simulink model "transversal_model"  (R2023b)
settings: Solver=FixedStepDiscrete  StartTime=0.0  StopTime=0.01  RelTol=1e-3
undefined symbols (not defined in the file): mf1, mf2, mf3, mfIdeal, pw
libraries: phaseddetectlib x9, phasedenvlib x4, phasedtxrxlib x2, dspfdesign x1, phasedwavlib x1
settings Model: Creator=krsh  LastModifiedBy=krsh
settings SolverCC: AlgebraicLoopSolver=TrustRegion  AutoInsertRateTranBlk=on
settings DataIOCC: LimitDataPoints=on  SaveOutput=off  SignalLogging=off  SaveTime=off
settings OptimizationCC: ReuseModelBlockBuffer=off  LifeSpan=inf  SimCompilerOptimization=on
settings DebuggingCC: AlgebraicLoopMsg=error  SingleTaskRateTransMsg=error  UnconnectedInputMsg=warning  UnconnectedOutputMsg=warning  UnconnectedLineMsg=warning  AllowSymbolicDim=off  SubsystemReferenceDiagnosticForUnitTest=warning  SFUnexpectedBacktrackingDiag=warning  SFNoUnconditionalDefaultTransitionDiag=warning  SFExecutionAtInitializationDiag=none  ArithmeticOperatorsInVariantConditions=warning
settings ModelReferenceCC: EnableRefExpFcnMdlSchedulingChecks=on
settings SFSimCC: SimUseLocalCustomCode=off  CustomCodeUndefinedFunction=UseInterfaceOnly
settings RTWCC: RTWUseLocalCustomCode=off
settings CodeAppCC: StateflowObjectComments=on
settings GRTTargetCC: TargetLangStandard=C89/C90 (ANSI)
settings ConfigComp: CovMetricSettings=dw  CovSaveCumulativeToWorkspaceVar=on  CovSaveSingleToWorkspaceVar=on  CovExternalEMLEnable=off  CovSFcnEnable=off

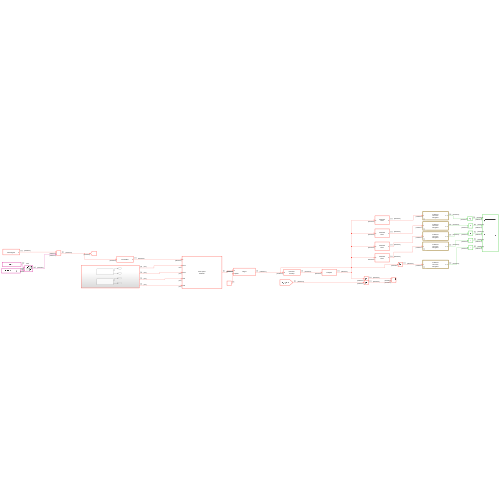
[thumbnail: Simulink's stored preview of the top-level diagram]
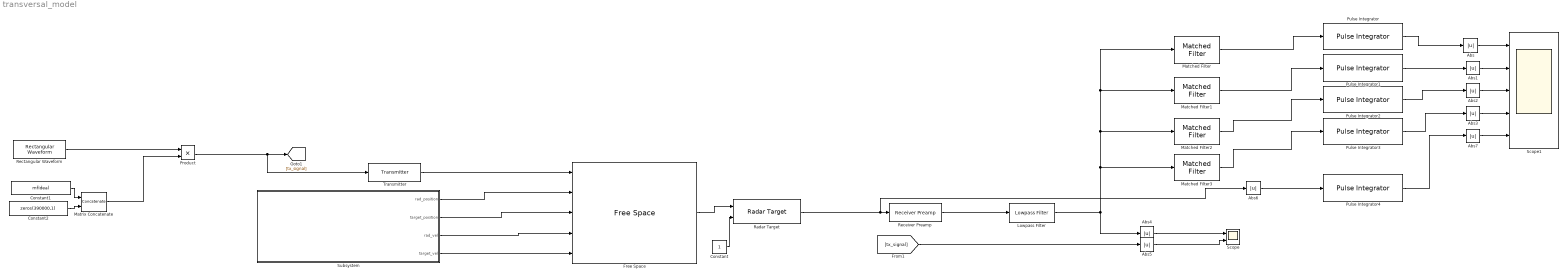
== system transversal_model ==
  Abs{,1..7} (8 alike) : Abs  SaturateOnIntegerOverflow=off
  Constant : Constant  SampleTime=-1
  Constant1 : Constant  Value=mfIdeal
  Constant2 : Constant  Value=zeros(390000,1)
  Free Space : phasedenvlib/Free Space  PropagationSpeed=c  OperatingFrequency=3e8  TwoWayPropagation=off  SampleRateFromInputCheckbox=on  SampleRate=1e6  MaximumDistanceSource=Property  MaximumDistance=2e3  MaximumNumInputSamplesSource=Auto  MaximumNumInputSamples=1000  SimulateUsing=Interpreted execution
  Lowpass Filter : dspfdesign/Lowpass Filter  FilterType=IIR  DesignForMinimumOrder=off  FilterOrder=3  PassbandFrequency=pulse_bw  StopbandFrequency=12e3  PassbandRipple=0.1  StopbandAttenuation=80  SampleRateMode=Specify on dialog  SampleRate=fs  SimulateUsing=Interpreted execution  roundingMode=Floor  coeffsDataTypeStr=fixdt(1,16)
  Matched Filter : phaseddetectlib/Matched Filter  CoefficientsSource=Property  Coefficients=mfIdeal'  SpectrumWindow=None  CustomSpectrumWindow=@hamming  SpectrumRange=[ 0, 1e5 ]  SampleRateFromInputCheckbox=on  SampleRate=1e6  SidelobeAttenuation=30  Beta=0.5  Nbar=4  GainOutputPort=off  MaximumNumInputSamplesSource=Auto  MaximumNumInputSamples=100  SimulateUsing=Interpreted execution
  Matched Filter1 : phaseddetectlib/Matched Filter  CoefficientsSource=Property  Coefficients=mf1.coeffs.Numerator'  SpectrumWindow=None  CustomSpectrumWindow=@hamming  SpectrumRange=[ 0, 1e5 ]  SampleRateFromInputCheckbox=on  SampleRate=1e6  SidelobeAttenuation=30  Beta=0.5  Nbar=4  GainOutputPort=off  MaximumNumInputSamplesSource=Auto  MaximumNumInputSamples=100  SimulateUsing=Interpreted execution
  Matched Filter2 : phaseddetectlib/Matched Filter  CoefficientsSource=Property  Coefficients=mf2.coeffs.Numerator'  SpectrumWindow=None  CustomSpectrumWindow=@hamming  SpectrumRange=[ 0, 1e5 ]  SampleRateFromInputCheckbox=on  SampleRate=1e6  SidelobeAttenuation=30  Beta=0.5  Nbar=4  GainOutputPort=off  MaximumNumInputSamplesSource=Auto  MaximumNumInputSamples=100  SimulateUsing=Interpreted execution
  Matched Filter3 : phaseddetectlib/Matched Filter  CoefficientsSource=Property  Coefficients=mf3.coeffs.Numerator'  SpectrumWindow=None  CustomSpectrumWindow=@hamming  SpectrumRange=[ 0, 1e5 ]  SampleRateFromInputCheckbox=on  SampleRate=1e6  SidelobeAttenuation=30  Beta=0.5  Nbar=4  GainOutputPort=off  MaximumNumInputSamplesSource=Auto  MaximumNumInputSamples=100  SimulateUsing=Interpreted execution
  Matrix Concatenate : Concatenate  Mode=Multidimensional array
  Product : Product
  Pulse Integrator{,1..4} (5 alike) : phaseddetectlib/Pulse Integrator  CoherentFlag=Coherent  N=10  V=0
  Radar Target : phasedenvlib/Radar Target  EnablePolarization=off  Mode=Monostatic  MeanRCSSource=Property  ScatteringMatrixSource=Property  MeanRCS=1  ScatteringMatrix=eye( 2 )  Model=Swerling1  PropagationSpeed=c  OperatingFrequency=3e8  SeedSource=Auto  Seed=0  SimulateUsing=Interpreted execution
  Receiver Preamp : phasedtxrxlib/Receiver Preamp  Gain=3  LossFactor=0  NoiseMethod=Noise power  NoiseFigure=1.2  ReferenceTemperature=290  SampleRateFromInputCheckbox=on  SampleRate=1e6  NoisePower=0.002  EnableInputPort=off  PhaseNoiseInputPort=off  SeedSource=Auto  Seed=0  SimulateUsing=Interpreted execution
  Rectangular Waveform : phasedwavlib/Rectangular Waveform  SampleRate=fs  DurationSpecification=Pulse width  PulseWidth=pw  DutyCycle=0.5  PRF=prf  PRFSelectionInputPort=off  SimulationTimeSource=Derive from waveform parameters  FrequencyOffsetSource=Property  FrequencyOffset=0  OutputFormat=Pulses  NumSamples=100  NumPulses=1  PRFOutputPort=off  CoefficientsOutputPort=off  SimulateUsing=Interpreted execution
  Scope : Scope  NumInputPorts=2
  Scope1 : Scope  NumInputPorts=5
  Subsystem : Subsystem
  Transmitter : phasedtxrxlib/Transmitter  PeakPower=tx_peak_power  Gain=13  LossFactor=0  InUseOutputPort=off  CoherentOnTransmit=on  PhaseNoiseOutputPort=off  SeedSource=Auto  Seed=0  SimulateUsing=Interpreted execution
  wires:
  Product/1 -> Transmitter/1, [tx_signal]
  Subsystem/1(rad_position) -> Free Space/2
  Subsystem/2(target_position) -> Free Space/3
  Subsystem/3(rad_vel) -> Free Space/4
  Subsystem/4(target_vel) -> Free Space/5
  Transmitter/1 -> Free Space/1
  [tx_signal] -> Abs5/1
  Free Space/1 -> Radar Target/1
  Constant/1 -> Radar Target/2
  Matched Filter/1 -> Pulse Integrator/1
  Matched Filter1/1 -> Pulse Integrator1/1
  Matched Filter2/1 -> Pulse Integrator2/1
  Matched Filter3/1 -> Pulse Integrator3/1
  Abs4/1 -> Scope/1
  Abs5/1 -> Scope/2
  Abs6/1 -> Pulse Integrator4/1
  Radar Target/1 -> Abs6/1, Receiver Preamp/1
  Receiver Preamp/1 -> Lowpass Filter/1
  Pulse Integrator/1 -> Abs/1
  Pulse Integrator1/1 -> Abs1/1
  Pulse Integrator2/1 -> Abs2/1
  Pulse Integrator3/1 -> Abs3/1
  Pulse Integrator4/1 -> Abs7/1
  Constant1/1 -> Matrix Concatenate/1
  Constant2/1 -> Matrix Concatenate/2
  Matrix Concatenate/1 -> Product/2
  Rectangular Waveform/1 -> Product/1
  Lowpass Filter/1 -> Matched Filter/1, Matched Filter1/1, Matched Filter2/1, Matched Filter3/1, Abs4/1
  Abs/1 -> Scope1/1
  Abs1/1 -> Scope1/2
  Abs2/1 -> Scope1/3
  Abs3/1 -> Scope1/4
  Abs7/1 -> Scope1/5

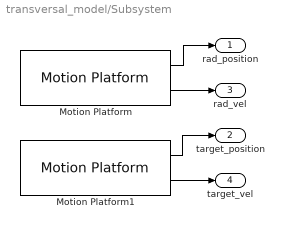
== system transversal_model/Subsystem ==
  Motion Platform : phasedenvlib/Motion Platform  MotionModel=Velocity  InitialPosition=[ 0; 0; 0 ]  InitialVelocity=[ 0; 0; 0 ]  VelocitySource=Property  Velocity=[0;0;0]  AccelerationSource=Property  Acceleration=[0;0;0]  CustomTrajectory=[ 0, 0, 0, 0, 0, 0, 0; 1, 0, 0, 0, 0, 0, 0 ]  ScanMode=None  InitialScanAngle=0  AzimuthSpan=[ -60, 60 ]  AzimuthScanRate=10  InitialOrientationAxes=eye( 3 )  OrientationAxesOutputPort=off  ElapsedTimeSource=Auto  SampleRateFromInputCheckbox=on  SampleRate=1e6  SimulateUsing=Interpreted execution
  Motion Platform1 : phasedenvlib/Motion Platform  MotionModel=Velocity  InitialPosition=[ 2000; 0; 0 ]  InitialVelocity=[ 0; 0; 0 ]  VelocitySource=Property  Velocity=[-100;0;0]  AccelerationSource=Property  Acceleration=[0;0;0]  CustomTrajectory=[ 0, 0, 0, 0, 0, 0, 0; 1, 0, 0, 0, 0, 0, 0 ]  ScanMode=None  InitialScanAngle=0  AzimuthSpan=[ -60, 60 ]  AzimuthScanRate=10  InitialOrientationAxes=eye( 3 )  OrientationAxesOutputPort=off  ElapsedTimeSource=Auto  SampleRateFromInputCheckbox=on  SampleRate=1e6  SimulateUsing=Interpreted execution
  rad_position : Outport
  target_position : Outport  Port=2
  rad_vel : Outport  Port=3
  target_vel : Outport  Port=4
  wires:
  Motion Platform1/2 -> target_vel/1
  Motion Platform1/1 -> target_position/1
  Motion Platform/2 -> rad_vel/1
  Motion Platform/1 -> rad_position/1
